simulink model "firdecimation_ref1"  (Simulink 4.00)
settings: Solver=FixedStepDiscrete  SolverMode=MultiTasking  StartTime=0.0  StopTime=30  RelTol=1e-3
PreLoadFcn:
  | load mtlb; whos mtlb Fs
PostLoadFcn:
  | set_param(gcs,'SimulationCommand','Update')
libraries: dspmlti3 x1, dspsrcs3 x1
settings Model: RequirementInfo=9  LastModifiedBy=dfass  LimitDataPoints=off  ExtModeTrigMode=oneshot  ExtModeArmWhenConnect=off  BlockReductionOpt=off

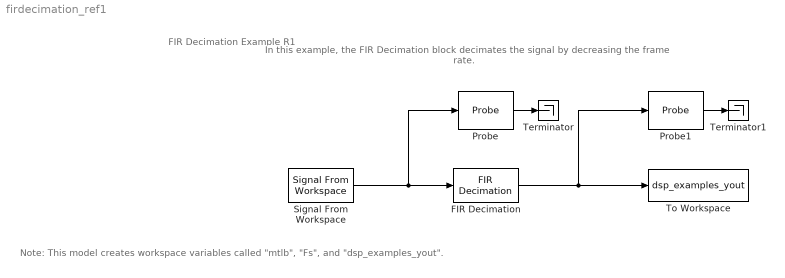
== system firdecimation_ref1 ==
  note: FIR Decimation Example R1
  note: In this example, the FIR Decimation block decimates the signal
      | by decreasing the frame rate.
  note: Note: This model creates workspace variables called "mtlb", "Fs", and "dsp_examples_yout".
  FIR Decimation : dspmlti3/FIR Decimation  h=fir1(35,0.4)  D=4  framing=Maintain input frame size
  Probe : Probe  ProbeWidth=off  ProbeSampleTime=on  ProbeComplexSignal=off  ProbeSignalDimensions=off
  Probe1 : Probe  ProbeWidth=off  ProbeSampleTime=on  ProbeComplexSignal=off  ProbeSignalDimensions=off
  Signal From Workspace : dspsrcs3/Signal From Workspace  X=mtlb  Ts=1/64  nsamps=64  OutputAfterFinalValue=Setting To Zero
  Terminator : Terminator
  Terminator1 : Terminator
  To Workspace : ToWorkspace  VariableName=dsp_examples_yout  SampleTime=-1  SaveFormat=Array
  wires:
  FIR Decimation/1 -> To Workspace/1, Probe1/1
  Signal From Workspace/1 -> Probe/1, FIR Decimation/1
  Probe/1 -> Terminator/1
  Probe1/1 -> Terminator1/1
